simulink model "testing"  (R2021a)
settings: Solver=VariableStepAuto  StartTime=0.0  StopTime=40  RelTol=1e-3
settings Model: Creator=shiva  LastModifiedBy=shiva

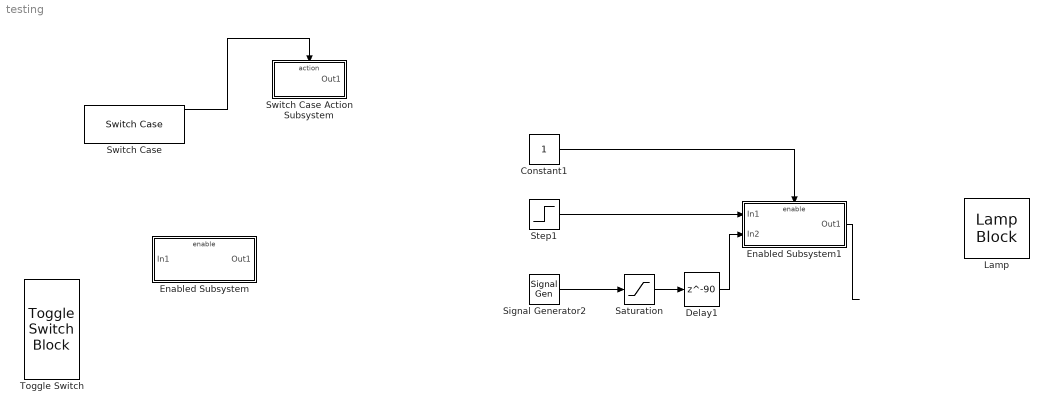
== system testing ==
  Constant1 : Constant
  Delay1 : Delay  DelayLength=90
  Enabled Subsystem : Subsystem  TreatAsAtomicUnit=on
  Enabled Subsystem1 : Subsystem  TreatAsAtomicUnit=on
  Lamp : LampBlock
  Saturation : Saturate  UpperLimit=1  LowerLimit=0
  Signal Generator2 : SignalGenerator  WaveForm=square
  Step1 : Step  Time=30  Before=1  After=0  SampleTime=0
  Switch Case : SwitchCase  CaseConditions={0,1,2,3}  ShowDefaultCase=off
  Switch Case Action Subsystem : Subsystem  TreatAsAtomicUnit=on
  Toggle Switch : ToggleSwitchBlock
      settings: Values={{'Off', 'On'}, [0 1]}
  wires:
  Step1/1 -> Enabled Subsystem1/1(In1)
  Constant1/1 -> Enabled Subsystem1/Enable
  Enabled Subsystem1/1(Out1) -> ?
  Saturation/1 -> Delay1/1
  Signal Generator2/1 -> Saturation/1
  Delay1/1 -> Enabled Subsystem1/2(In2)
  Switch Case/1 -> Switch Case Action Subsystem/Action

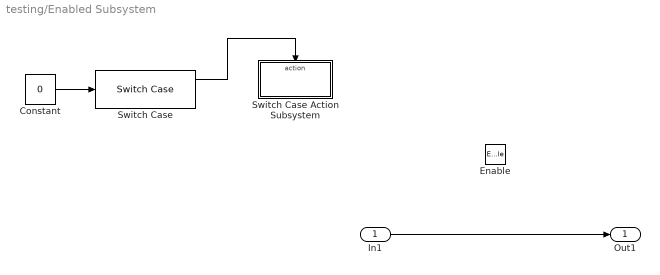
== system testing/Enabled Subsystem ==
  In1 : Inport
  Enable : EnablePort
  Constant : Constant  Value=0
  Switch Case : SwitchCase  CaseConditions={0,1}  ShowDefaultCase=off
  Switch Case Action Subsystem : Subsystem  TreatAsAtomicUnit=on
  Out1 : Outport
  wires:
  In1/1 -> Out1/1
  Constant/1 -> Switch Case/1
  Switch Case/1 -> Switch Case Action Subsystem/Action

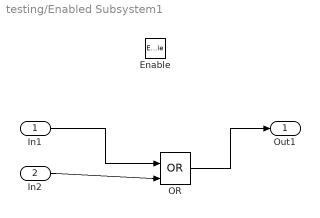
== system testing/Enabled Subsystem1 ==
  In1 : Inport
  In2 : Inport  Port=2
  Enable : EnablePort
  OR : Logic  Operator=OR  IconShape=distinctive  AllPortsSameDT=off  OutDataTypeStr=boolean
  Out1 : Outport
  wires:
  In1/1 -> OR/1
  In2/1 -> OR/2
  OR/1 -> Out1/1

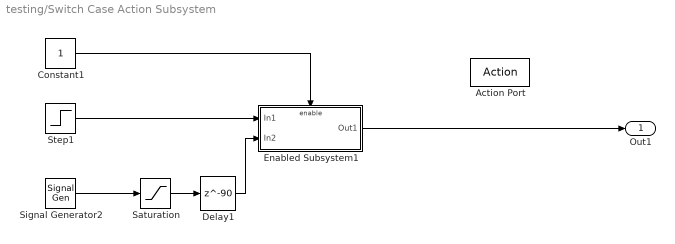
== system testing/Switch Case Action Subsystem ==
  Action Port : ActionPort  ActionPortLabel=case [ 0 ]:
  Constant1 : Constant
  Delay1 : Delay  DelayLength=90
  Enabled Subsystem1 : Subsystem  TreatAsAtomicUnit=on
  Saturation : Saturate  UpperLimit=1  LowerLimit=0
  Signal Generator2 : SignalGenerator  WaveForm=square
  Step1 : Step  Time=30  Before=1  After=0  SampleTime=0
  Out1 : Outport
  wires:
  Enabled Subsystem1/1(Out1) -> Out1/1
  Constant1/1 -> Enabled Subsystem1/Enable
  Signal Generator2/1 -> Saturation/1
  Delay1/1 -> Enabled Subsystem1/2(In2)
  Step1/1 -> Enabled Subsystem1/1(In1)
  Saturation/1 -> Delay1/1

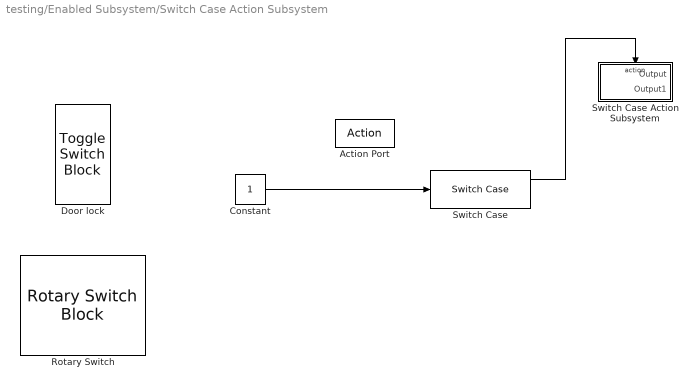
== system testing/Enabled Subsystem/Switch Case Action Subsystem ==
  Action Port : ActionPort  ActionPortLabel=case [ 0 ]:
  Constant : Constant
  Door lock : ToggleSwitchBlock
      settings: Values={{'Off', 'On'}, [0 1]}
  Rotary Switch : RotarySwitchBlock
      settings: Values={{'single press', 'double press'}, [0 1]}
  Switch Case : SwitchCase  CaseConditions={0,1}  ShowDefaultCase=off
  Switch Case Action Subsystem : Subsystem  TreatAsAtomicUnit=on
  wires:
  Constant/1 -> Switch Case/1
  Switch Case/1 -> Switch Case Action Subsystem/Action

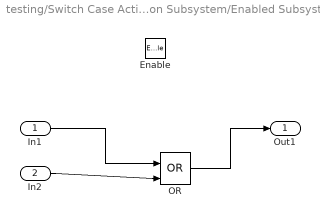
== system testing/Switch Case Action Subsystem/Enabled Subsystem1 ==
  In1 : Inport
  In2 : Inport  Port=2
  Enable : EnablePort
  OR : Logic  Operator=OR  IconShape=distinctive  AllPortsSameDT=off  OutDataTypeStr=boolean
  Out1 : Outport
  wires:
  In1/1 -> OR/1
  In2/1 -> OR/2
  OR/1 -> Out1/1

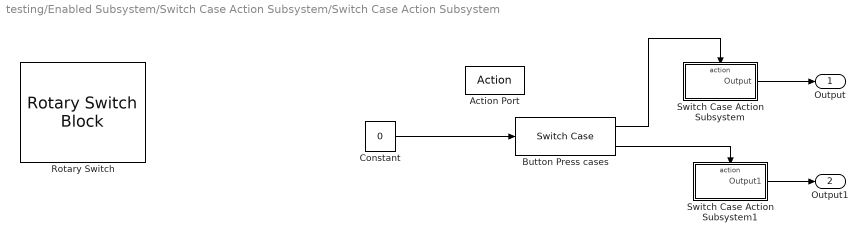
== system testing/Enabled Subsystem/Switch Case Action Subsystem/Switch Case Action Subsystem ==
  Action Port : ActionPort  ActionPortLabel=case [ 0 ]:
  Button Press cases : SwitchCase  CaseConditions={0,1}  ShowDefaultCase=off
  Constant : Constant  Value=0
  Rotary Switch : RotarySwitchBlock
      settings: Values={{'single press', 'double press'}, [0 1]}
  Switch Case Action Subsystem : Subsystem  TreatAsAtomicUnit=on
  Switch Case Action Subsystem1 : Subsystem  TreatAsAtomicUnit=on
  Output : Outport
  Output1 : Outport  Port=2
  wires:
  Constant/1 -> Button Press cases/1
  Button Press cases/1 -> Switch Case Action Subsystem/Action
  Button Press cases/2 -> Switch Case Action Subsystem1/Action
  Switch Case Action Subsystem/1(Output) -> Output/1
  Switch Case Action Subsystem1/1(Output1) -> Output1/1

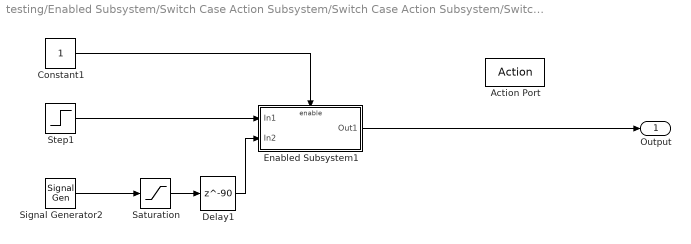
== system testing/Enabled Subsystem/Switch Case Action Subsystem/Switch Case Action Subsystem/Switch Case Action Subsystem ==
  Action Port : ActionPort  ActionPortLabel=case [ 0 ]:
  Constant1 : Constant
  Delay1 : Delay  DelayLength=90
  Enabled Subsystem1 : Subsystem  TreatAsAtomicUnit=on
  Saturation : Saturate  UpperLimit=1  LowerLimit=0
  Signal Generator2 : SignalGenerator  WaveForm=square
  Step1 : Step  Time=30  Before=1  After=0  SampleTime=0
  Output : Outport
  wires:
  Enabled Subsystem1/1(Out1) -> Output/1
  Constant1/1 -> Enabled Subsystem1/Enable
  Signal Generator2/1 -> Saturation/1
  Delay1/1 -> Enabled Subsystem1/2(In2)
  Step1/1 -> Enabled Subsystem1/1(In1)
  Saturation/1 -> Delay1/1

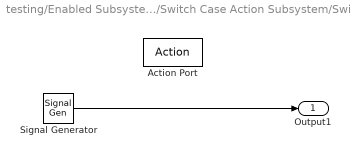
== system testing/Enabled Subsystem/Switch Case Action Subsystem/Switch Case Action Subsystem/Switch Case Action Subsystem1 ==
  Action Port : ActionPort  ActionPortLabel=case [ 1 ]:
  Signal Generator : SignalGenerator  Frequency=0.0005  Units=rad/sec
  Output1 : Outport
  wires:
  Signal Generator/1 -> Output1/1

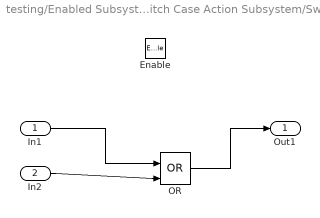
== system testing/Enabled Subsystem/Switch Case Action Subsystem/Switch Case Action Subsystem/Switch Case Action Subsystem/Enabled Subsystem1 ==
  In1 : Inport
  In2 : Inport  Port=2
  Enable : EnablePort
  OR : Logic  Operator=OR  IconShape=distinctive  AllPortsSameDT=off  OutDataTypeStr=boolean
  Out1 : Outport
  wires:
  In1/1 -> OR/1
  In2/1 -> OR/2
  OR/1 -> Out1/1
